simulink model "accBasedController_Simulation"  (R2020a)
settings: Solver=VariableStepAuto  StartTime=0  StopTime=20  FixedStep=0.001  RelTol=1e-3
values from neighbouring files (symbols this model uses):
  A = [0 0 5.53191489362 0 0 0 0 -107.82412766 0 221.276595745 0 1 ... (25 elements, 5x5)]    [CACu_ws.mat]    (also in SimulationParameters.m = [0 0 0 1 0 0;      0 0 0 0 1 0;      0 0 0 0 0 1;      -Ka/J; Simulation_ws.mat = [0 0 0 -118.993135011 5.87581816357 0 0 0 0 118.993135011 -1; abc_ws.mat = [0 0 0 1828.84460673 0 0 0 0 -1965.91569285 221.276595745 0 ; kalmanSS.m = [0 0 0 1 0 0;      0 0 0 0 1 0;      0 0 0 0 0 1;      -Ka/J)
  B = [1  0; 0  0; 0  0; 0  0; 0  19.2446808511]    [CACu_ws.mat]    (also in SimulationParameters.m = [zeros(3,control_dim); 1/Jh 0 0; 0 -1/Je 0; 0 0 N*KI/Ja]; Simulation_ws.mat = [0 0 0 22.8832951945 0 0 0 0 0 0 -1.12996503145 0 ... (18 el; abc_ws.mat = [1 0 0 0 0 0 0 0 -1.31799121269 0 0 0 ... (15 elements, 5x3); kalmanSS.m = [zeros(3,control_dim); 1/Jh 0 0; 0 -1/Je 0; 0 0 N*KI/Ja])
  C = [0 0 0 0 0 0 1 0 0 0 0 0 ... (25 elements, 5x5)]    [CACu_ws.mat]    (also in SimulationParameters.m = [zeros(sensor_dim,state_dim)]; Simulation_ws.mat = [-5.2 0 0 0 0 0 5.2 0 1 0 0 0 ... (36 elements, 6x6)]; abc_ws.mat; kalmanSS.m = [zeros(sensor_dim,state_dim)])
  CURRENT_MAX = 3.14    [CAC_ws.mat]    (also in CACu_ws.mat; SimulationParameters.m = 3.14159265359; Simulation_ws.mat = 3.14159265359; TransferFunctions.m = 3.14159265359)
  D = [1  0; 0  0; 0  0; 0  0; 0  0]    [CACu_ws.mat]    (also in SimulationParameters.m = zeros(sensor_dim, control_dim); Simulation_ws.mat = [0 0 0 0 0 0 0 0 0 0 0 0 ... (18 elements, 6x3)]; abc_ws.mat = [1 0 0 0 0 0 0 0 0 0 0 0 ... (15 elements, 5x3)]; kalmanSS.m = zeros(sensor_dim, control_dim))
  damping_d = 1.6    [CAC_ws.mat]    (also in CACu_ws.mat = 0.770835010154; abc_ws.mat = 0.770835010154; kalmanSSHumInput.m = 0.9; kalmanStateSpaceModellingHumInput.m = 0.9)
  dt = 0.001    [SimulationParameters.m]    (also in Simulation_ws.mat; TransferFunctions.m; kalmanSS.m; tests_analysis.m = 0.008)
  epos_Ki = 1.19    [CAC_ws.mat]    (also in CACu_ws.mat; TransferFunctions.m; abc_ws.mat; kalmanSSHumInput.m)
  epos_Kp = 11.9    [CAC_ws.mat]    (also in CACu_ws.mat; TransferFunctions.m; abc_ws.mat; kalmanSSHumInput.m)
  Fk = eye(state_dim) + A*dt + (A*dt)^2/prod(1:2) + (A*dt)^3/prod(1:3) + (A*dt)^4/prod(1:4)    [SimulationParameters.m]    (also in Simulation_ws.mat = [0.999940504052 2.93784973961e-06 5.41742100187e-11 -0.11899; kalmanSS.m)
  Gk = dt*(eye(state_dim) + A*dt/prod(1:2) + (A*dt)^2/prod(1:3) + (A*dt)^3/prod(1:4) +         (A*dt)^4/prod(1:5))*B    [SimulationParameters.m]    (also in Simulation_ws.mat = [1.14415341408e-05 5.60242006442e-12 0 0.0228828413715 2.240; kalmanSS.m = dt*(eye(state_dim) + A*dt/prod(1:2) + (A*dt)^2/prod(1:3) + ()
  I_zz = mass_scale*body_mass*(L_leg*r_zz)^2    (= 0.0437446334976)    [KneeJointParameters.m]    (also in SimulationParameters.m; Simulation_ws.mat; TransferFunctions.m; abc_ws.mat)
  Ja = 0.47    [CACu_ws.mat]    (also in SimulationParameters.m; Simulation_ws.mat; TransferFunctions.m; abc_ws.mat)
  Je = 0.94    [CACu_ws.mat]    (also in SimulationParameters.m = 0.88498313856; Simulation_ws.mat = 0.88498313856; TransferFunctions.m = 0.88498313856; abc_ws.mat = 0.7587304)
  Jh = 0.05    [CACu_ws.mat]    (also in SimulationParameters.m = 0.0437; Simulation_ws.mat = 0.0437; TransferFunctions.m = 0.0437; abc_ws.mat = 0.0437)
  Ka = 5.2    [CACu_ws.mat]    (also in SimulationParameters.m; Simulation_ws.mat; TransferFunctions.m = 6552; abc_ws.mat = 1387.6)
  KI = 0.0603    [CACu_ws.mat]    (also in SimulationParameters.m; Simulation_ws.mat; TransferFunctions.m; abc_ws.mat)
  Ks = 104    [CACu_ws.mat]    (also in SimulationParameters.m; Simulation_ws.mat; TransferFunctions.m; abc_ws.mat)
  Le = 0.4    [CACu_ws.mat]    (also in SimulationParameters.m = 0.432; Simulation_ws.mat = 0.432; TransferFunctions.m = 0.432; abc_ws.mat)
  N = 150    [CACu_ws.mat]    (also in SimulationParameters.m; Simulation_ws.mat; TransferFunctions.m; abc_ws.mat)
  Rk = eye(sensor_dim)    [kalmanStateSpaceModellingWithoutHum.m]
  sensor_dim = 5    [CACu_ws.mat]    (also in SimulationParameters.m = 6; Simulation_ws.mat = 6; abc_ws.mat; kalmanSS.m = 6)
  state_dim = 5    [CACu_ws.mat]    (also in SimulationParameters.m = 6; Simulation_ws.mat = 6; abc_ws.mat; kalmanSS.m = 6)
  stiffness_d = 1.04    [CAC_ws.mat]    (also in CACu_ws.mat = 14.0803237251; abc_ws.mat = 14.0803237251; kalmanSSHumInput.m = 3.874; kalmanStateSpaceModellingHumInput.m = 3.874)
  stiffness_lower = -20.9019922533    [CACu_ws.mat]    (also in abc_ws.mat; kalmanSSHumInput.m = -24.4873189611; kalmanStateSpaceModellingHumInput.m = -24.4873189611)
  Threaded_Ts = 0.001    [CAC_ws.mat]    (also in CACu_ws.mat; SimulationParameters.m; Simulation_ws.mat; abc_ws.mat)
  We = 19.6133    [CACu_ws.mat]    (also in SimulationParameters.m = 46.5037717323; Simulation_ws.mat = 46.5037717323; TransferFunctions.m = 46.5037717323; abc_ws.mat = 46.5037717323)
  zeta = 0.06    [SimulationParameters.m]    (also in Simulation_ws.mat; TransferFunctions.m; abc_ws.mat; kalmanSSHumInput.m = 0.01)
undefined symbols (not defined in the file or in its folder): A_kf, alpha, B_kf, C_kf, Continuous, D_kf, DiscIntNeverNeededParam, Discrete, gamma, k_bar, kf_ste_dim, nm_window, p_e_idx, p_m_idx, rho, sigma, Time, v_e_idx, v_h_idx, v_m_idx
libraries: simulink x23, dspstat3 x8, simulink_extras x5, ctrlSharedLib x2, dspsigops x2
(part 2 of 2)

== system accBasedController_Simulation/Secantes ==
  rms : Inport
  Trigger : TriggerPort  VariantControl=Variant
  Constant : Constant  Value=0.853
  Constant1 : Constant  Value=170
  Constant2 : Constant  Value=200
  Constant3 : Constant  Value=1.040
  Delay{,1..3} (4 alike) : Delay  DelayLength=1  InitialConditionSource=Input port
      settings: InputPortMap=u0,p4
  Divide : Product  Inputs=*/
  Product : Product
  Saturation : Saturate  UpperLimit=500  LowerLimit=0
  Sum : Sum  Inputs=+-
  Sum1 : Sum  Inputs=|-+
  Sum2 : Sum  Inputs=|+-
  Kp_new : Outport
  wires:
  rms/1 -> Delay3/1
  Constant/1 -> Delay/2
  Delay/1 -> Sum/2
  Product/1 -> Sum1/1
  Saturation/1 -> Delay1/1, Kp_new/1
  Constant1/1 -> Delay1/2
  Delay1/1 -> Delay2/1, Sum2/1, Sum1/2
  Divide/1 -> Product/2
  Sum/1 -> Divide/2
  Sum2/1 -> Divide/1
  Constant2/1 -> Delay2/2
  Constant3/1 -> Delay3/2
  Delay3/1 -> Delay/1, Sum/1, Product/1
  Delay2/1 -> Sum2/2
  Sum1/1 -> Saturation/1

== system accBasedController_Simulation/Subsystem ==
  x : Inport
  Constant12 : Constant  Value=1/dt
  Constant13 : Constant  Value=7
  Gain17 : Gain  Gain=1/(dt)
  LowPassFilter2p : Subsystem
  Sum : Sum  Inputs=|+-
  Unit Delay1 : UnitDelay  SampleTime=-1  HasFrameUpgradeWarning=on
  dot_x : Outport
  wires:
  Unit Delay1/1 -> Sum/2
  Sum/1 -> Gain17/1
  Gain17/1 -> LowPassFilter2p/1(sample)
  LowPassFilter2p/1(output) -> dot_x/1
  Constant12/1 -> LowPassFilter2p/3(sample_freq)
  x/1 -> Unit Delay1/1, Sum/1
  Constant13/1 -> LowPassFilter2p/2(cutoff_freq)

== system accBasedController_Simulation/Subsystem1 ==
  x : Inport
  Constant12 : Constant  Value=1/dt
  Constant13 : Constant  Value=7
  Gain17 : Gain  Gain=1/(dt)
  LowPassFilter2p : Subsystem
  Sum : Sum  Inputs=|+-
  Unit Delay1 : UnitDelay  SampleTime=-1  HasFrameUpgradeWarning=on
  dot_x : Outport
  wires:
  Constant13/1 -> LowPassFilter2p/2(cutoff_freq)
  x/1 -> Sum/1, Unit Delay1/1
  Constant12/1 -> LowPassFilter2p/3(sample_freq)
  LowPassFilter2p/1(output) -> dot_x/1
  Gain17/1 -> LowPassFilter2p/1(sample)
  Sum/1 -> Gain17/1
  Unit Delay1/1 -> Sum/2

== system accBasedController_Simulation/Subsystem2 ==
  x : Inport
  Constant12 : Constant  Value=1/dt
  Constant13 : Constant  Value=5
  Gain17 : Gain  Gain=1/(dt)
  LowPassFilter2p : Subsystem
  Sum : Sum  Inputs=|+-
  Unit Delay1 : UnitDelay  SampleTime=-1  HasFrameUpgradeWarning=on
  dot_x : Outport
  wires:
  Constant13/1 -> LowPassFilter2p/2(cutoff_freq)
  x/1 -> Sum/1, Unit Delay1/1
  Constant12/1 -> LowPassFilter2p/3(sample_freq)
  LowPassFilter2p/1(output) -> dot_x/1
  Gain17/1 -> LowPassFilter2p/1(sample)
  Sum/1 -> Gain17/1
  Unit Delay1/1 -> Sum/2

== system accBasedController_Simulation/UnitDelay ==
  In1 : Inport
  Unit Delay : UnitDelay  SampleTime=-1  HasFrameUpgradeWarning=on
  y : Outport  VectorParamsAs1DForOutWhenUnconnected=off
  wires:
  Unit Delay/1 -> y/1
  In1/1 -> Unit Delay/1

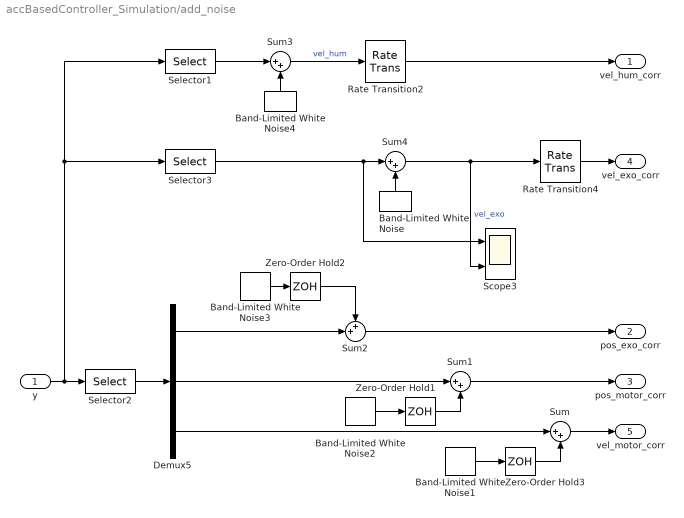
== system accBasedController_Simulation/add_noise ==
  y : Inport
  Band-Limited White Noise : simulink/Sources/Band-Limited White Noise  Cov=5.476e-6  Ts=dt  seed=[23341]  VectorParams1D=off
  Band-Limited White Noise1 : simulink/Sources/Band-Limited White Noise  Cov=1.096e-2  Ts=dt  seed=[23541]  VectorParams1D=off
  Band-Limited White Noise2 : simulink/Sources/Band-Limited White Noise  Cov=2.353e-6  Ts=dt  seed=[23543]  VectorParams1D=off
  Band-Limited White Noise3 : simulink/Sources/Band-Limited White Noise  Cov=9.412e-6  Ts=dt  seed=[87541]  VectorParams1D=off
  Band-Limited White Noise4 : simulink/Sources/Band-Limited White Noise  Cov=5.476e-6  Ts=dt  seed=[41236]  VectorParams1D=off
  Demux5 : Demux  Outputs=3
  Rate Transition2 : RateTransition  OutPortSampleTime=0.008
  Rate Transition4 : RateTransition  OutPortSampleTime=0.008
  Scope3 : Scope  NumInputPorts=2
  Selector1 : Selector  InputPortWidth=sensor_dim  IndexOptions=Index vector (dialog)  Indices=[v_h_idx]  OutputSizes=1
  Selector2 : Selector  InputPortWidth=sensor_dim  IndexOptions=Index vector (dialog)  Indices=[p_e_idx, p_m_idx, v_m_idx]  OutputSizes=1
  Selector3 : Selector  InputPortWidth=sensor_dim  IndexOptions=Index vector (dialog)  Indices=[v_e_idx]  OutputSizes=1
  Sum{,1,3..4} (4 alike) : Sum  Inputs=|++
  Sum2 : Sum  Inputs=++|
  Zero-Order Hold1 : ZeroOrderHold  SampleTime=dt
  Zero-Order Hold2 : ZeroOrderHold  SampleTime=dt
  Zero-Order Hold3 : ZeroOrderHold  SampleTime=dt
  vel_hum_corr : Outport
  pos_exo_corr : Outport  Port=2
  pos_motor_corr : Outport  Port=3
  vel_exo_corr : Outport  Port=4
  vel_motor_corr : Outport  Port=5
  wires:
  Selector2/1 -> Demux5/1
  Sum/1 -> vel_motor_corr/1
  Demux5/3 -> Sum/1
  Zero-Order Hold3/1 -> Sum/2
  y/1 -> Selector3/1, Selector1/1, Selector2/1
  Band-Limited White Noise1/1 -> Zero-Order Hold3/1
  Band-Limited White Noise2/1 -> Zero-Order Hold1/1
  Zero-Order Hold1/1 -> Sum1/2
  Sum1/1 -> pos_motor_corr/1
  Demux5/2 -> Sum1/1
  Band-Limited White Noise3/1 -> Zero-Order Hold2/1
  Sum2/1 -> pos_exo_corr/1
  Demux5/1 -> Sum2/2
  Zero-Order Hold2/1 -> Sum2/1
  Band-Limited White Noise4/1 -> Sum3/2
  Selector1/1 -> Sum3/1
  Sum3/1 -> Rate Transition2/1  "vel_hum"
  Rate Transition2/1 -> vel_hum_corr/1
  Selector3/1 -> Sum4/1, Scope3/1
  Sum4/1 -> Rate Transition4/1, Scope3/2  "vel_exo"
  Band-Limited White Noise/1 -> Sum4/2
  Rate Transition4/1 -> vel_exo_corr/1

== system accBasedController_Simulation/noise_resample_filtering ==
  vel_hum : Inport
  vel_exo : Inport  Port=2
  Band-Limited White Noise : simulink/Sources/Band-Limited White Noise  Cov=[dt*dt*0.3]  Ts=dt  seed=[23341]  VectorParams1D=off
  Band-Limited White Noise1 : simulink/Sources/Band-Limited White Noise  Cov=[dt*dt*0.3]  Ts=dt  seed=[41236]  VectorParams1D=off
  LowPassFilter2p : Subsystem
  LowPassFilter2p1 : Subsystem
  Rate Transition2 : RateTransition  OutPortSampleTime=0.008
  Rate Transition4 : RateTransition  OutPortSampleTime=0.008
  Scope3 : Scope  NumInputPorts=3
  Sum1 : Sum  Inputs=|++
  Sum2 : Sum  Inputs=|++
  XSENS_FC : Constant  Value=60
  XSENS_FC1 : Constant  Value=60
  XSENS_RATE : Constant  Value=120
  XSENS_RATE1 : Constant  Value=120
  ve_hum_filt : Outport
  vel_exo_filt : Outport  Port=2
  wires:
  vel_hum/1 -> Sum2/1
  XSENS_FC/1 -> LowPassFilter2p/2(cutoff_freq)
  LowPassFilter2p/1(output) -> ve_hum_filt/1  "vel_hum"
  XSENS_FC1/1 -> LowPassFilter2p1/2(cutoff_freq)
  Rate Transition4/1 -> LowPassFilter2p1/1(sample)
  vel_exo/1 -> Scope3/1, Sum1/1
  LowPassFilter2p1/1(output) -> vel_exo_filt/1, Scope3/3
  Sum2/1 -> Rate Transition2/1  "vel_hum"
  Sum1/1 -> Scope3/2, Rate Transition4/1  "vel_exo"
  Band-Limited White Noise1/1 -> Sum2/2
  Rate Transition2/1 -> LowPassFilter2p/1(sample)
  XSENS_RATE/1 -> LowPassFilter2p/3(sample_freq)
  Band-Limited White Noise/1 -> Sum1/2
  XSENS_RATE1/1 -> LowPassFilter2p1/3(sample_freq)

== system accBasedController_Simulation/update_Ki ==
  Kp_acc : Inport
  zeta : Inport  Port=2
  Bias : Bias  Bias=Je
  Gain2 : Gain  Gain=Ka
  Gain3 : Gain  Gain=2
  Product : Product
  Sqrt1 : Sqrt  SaturateOnIntegerOverflow=on
  Ki_acc : Outport
  wires:
  Bias/1 -> Gain2/1
  Gain2/1 -> Sqrt1/1
  Gain3/1 -> Ki_acc/1
  Kp_acc/1 -> Bias/1
  Sqrt1/1 -> Product/1
  Product/1 -> Gain3/1
  zeta/1 -> Product/2

== system accBasedController_Simulation/update_Kp ==
  w_n : Inport
  Constant : Constant  Value=Ka
  Divide : Product  Inputs=*/
  Gain1 : Gain  Gain=Je
  Square : Math  Operator=square  SaturateOnIntegerOverflow=on
  Sum : Sum  Inputs=|+-
  Kp_acc : Outport
  wires:
  Divide/1 -> Kp_acc/1
  Sum/1 -> Divide/1
  w_n/1 -> Square/1
  Constant/1 -> Sum/1
  Gain1/1 -> Sum/2
  Square/1 -> Divide/2, Gain1/1

== system accBasedController_Simulation/AccBasedController/A(z) ==
  In1 : Inport
  A(s) : TransferFcn  Numerator=[k_bar 0]  Denominator=[damping_d stiffness_d]
  Rate Transition1 : RateTransition  OutPortSampleTime=0.001
  Zero-Order Hold : ZeroOrderHold  SampleTime=-1
  Out1 : Outport
  wires:
  Zero-Order Hold/1 -> A(s)/1
  A(s)/1 -> Rate Transition1/1
  In1/1 -> Zero-Order Hold/1
  Rate Transition1/1 -> Out1/1

== system accBasedController_Simulation/AccBasedController/Filtering1 ==
  note: // get_filt_alpha - calculate a filter alpha
      | float AC_PID::get_filt_alpha(float filt_hz) const
      | {
      |     if (is_zero(filt_hz)) {
      |         return 1.0f;
      |     }
      |
      |     // calculate alpha
      |     float rc = 1 / (M_2PI * filt_hz);
      |     return _dt / (_dt + rc);
      | }
  note: e.g.:
      |
      | _target += get_filt_T_alpha() * (target - _target);
  new : Inport
  cutoff_freq [Hz] : Inport  Port=2
  reset_filter : Inport  Port=3
  dt : Inport  Port=4
  Constant6 : Constant
  Memory4 : Memory  InheritSampleTime=on
  Mux : Mux  Inputs=2
  Product5 : Product
  Subtract6 : Sum  Inputs=+-
  Subtract7 : Sum
  Switch : Switch  Criteria=u2 ~= 0
  Switch1 : Switch  Criteria=u2 ~= 0
  alpha : Fcn  Expr=u(1)/(u(1)+1/(2*pi*u(2)))
  filtered : Outport
  wires:
  Subtract7/1 -> Switch1/3
  Switch1/1 -> Memory4/1, filtered/1
  reset_filter/1 -> Switch1/2
  [alpha] -> Product5/1
  Switch/1 -> [alpha]
  Constant6/1 -> Switch/3
  new/1 -> Subtract6/1, Switch1/1
  Memory4/1 -> Subtract6/2, Subtract7/2
  Subtract6/1 -> Product5/2
  Product5/1 -> Subtract7/1
  Mux/1 -> alpha/1
  cutoff_freq [Hz]/1 -> Switch/2, Mux/2
  alpha/1 -> Switch/1
  dt/1 -> Mux/1

== system accBasedController_Simulation/AccBasedController/Filtering2 ==
  note: e.g.:
      |
      | _target += get_filt_T_alpha() * (target - _target);
  note: // get_filt_alpha - calculate a filter alpha
      | float AC_PID::get_filt_alpha(float filt_hz) const
      | {
      |     if (is_zero(filt_hz)) {
      |         return 1.0f;
      |     }
      |
      |     // calculate alpha
      |     float rc = 1 / (M_2PI * filt_hz);
      |     return _dt / (_dt + rc);
      | }
  new : Inport
  cutoff_freq [Hz] : Inport  Port=2
  reset_filter : Inport  Port=3
  dt : Inport  Port=4
  Constant6 : Constant
  Memory4 : Memory  InheritSampleTime=on
  Mux : Mux  Inputs=2
  Product5 : Product
  Subtract6 : Sum  Inputs=+-
  Subtract7 : Sum
  Switch : Switch  Criteria=u2 ~= 0
  Switch1 : Switch  Criteria=u2 ~= 0
  alpha : Fcn  Expr=u(1)/(u(1)+1/(2*pi*u(2)))
  filtered : Outport
  wires:
  dt/1 -> Mux/1
  alpha/1 -> Switch/1
  cutoff_freq [Hz]/1 -> Mux/2, Switch/2
  Mux/1 -> alpha/1
  Product5/1 -> Subtract7/1
  Subtract6/1 -> Product5/2
  Memory4/1 -> Subtract7/2, Subtract6/2
  new/1 -> Switch1/1, Subtract6/1
  Constant6/1 -> Switch/3
  Switch/1 -> [alpha]
  [alpha] -> Product5/1
  reset_filter/1 -> Switch1/2
  Switch1/1 -> filtered/1, Memory4/1
  Subtract7/1 -> Switch1/3

== system accBasedController_Simulation/AccBasedController/update_Ki ==
  Kp_acc : Inport
  Bias : Bias  Bias=Je
  Gain2 : Gain  Gain=Ka
  Gain3 : Gain  Gain=2*zeta
  Sqrt1 : Sqrt  SaturateOnIntegerOverflow=on
  Ki_acc : Outport
  wires:
  Sqrt1/1 -> Gain3/1
  Bias/1 -> Gain2/1
  Gain2/1 -> Sqrt1/1
  Gain3/1 -> Ki_acc/1
  Kp_acc/1 -> Bias/1

== system accBasedController_Simulation/AccBasedController/update_Kp ==
  w_n_sq : Inport
  Constant : Constant  Value=Ka
  Divide : Product  Inputs=*/
  Gain1 : Gain  Gain=Je
  Sum : Sum  Inputs=|+-
  Kp_acc : Outport
  wires:
  Divide/1 -> Kp_acc/1
  Sum/1 -> Divide/1
  w_n_sq/1 -> Divide/2, Gain1/1
  Constant/1 -> Sum/1
  Gain1/1 -> Sum/2

== system accBasedController_Simulation/AccBasedController/w_n_desired ==
  KneePosition : Inport
  Gain2 : Gain  Gain=1/I_zz
  k0 : Bias  Bias=110.0
  k1 : Gain  Gain=169.3
  w_n_sq : Outport
  wires:
  KneePosition/1 -> k1/1
  k1/1 -> k0/1
  Gain2/1 -> w_n_sq/1
  k0/1 -> Gain2/1  "K_j"

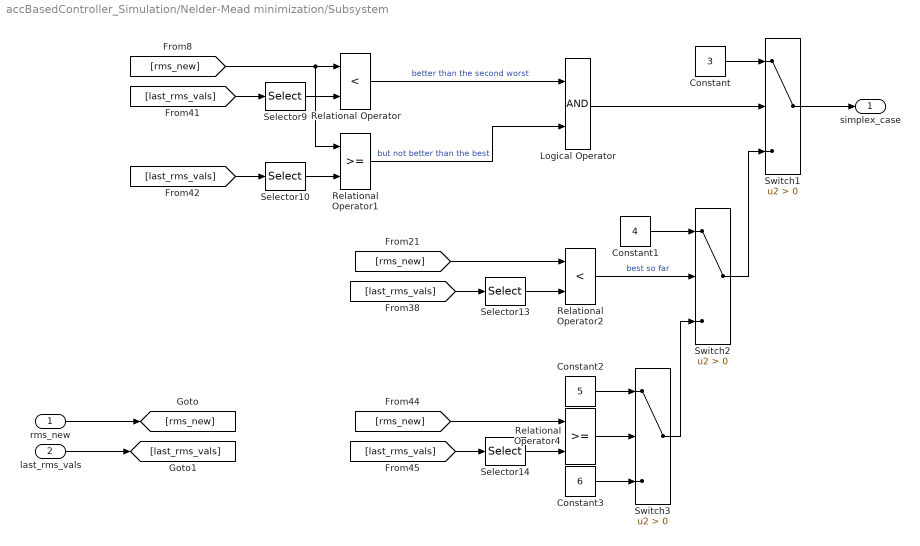
== system accBasedController_Simulation/Nelder-Mead minimization/Subsystem ==
  rms_new : Inport
  last_rms_vals : Inport  Port=2
  Constant : Constant  Value=3
  Constant1 : Constant  Value=4
  Constant2 : Constant  Value=5
  Constant3 : Constant  Value=6
  Logical Operator : Logic  AllPortsSameDT=off  OutDataTypeStr=boolean
  Relational Operator : RelationalOperator  Operator=<  OutDataTypeStr=boolean  RndMeth=Simplest
  Relational Operator1 : RelationalOperator  OutDataTypeStr=boolean  RndMeth=Simplest
  Relational Operator2 : RelationalOperator  Operator=<  OutDataTypeStr=boolean  RndMeth=Simplest
  Relational Operator4 : RelationalOperator  OutDataTypeStr=boolean  RndMeth=Simplest
  Selector10 : Selector  InputPortWidth=3  IndexOptions=Index vector (dialog)  Indices=[1]  OutputSizes=1
  Selector13 : Selector  InputPortWidth=3  IndexOptions=Index vector (dialog)  Indices=[1]  OutputSizes=1
  Selector14 : Selector  InputPortWidth=3  IndexOptions=Index vector (dialog)  Indices=[2]  OutputSizes=1
  Selector9 : Selector  InputPortWidth=3  IndexOptions=Index vector (dialog)  Indices=[2]  OutputSizes=1
  Switch1 : Switch  Criteria=u2 > Threshold
  Switch2 : Switch  Criteria=u2 > Threshold
  Switch3 : Switch  Criteria=u2 > Threshold
  simplex_case : Outport
  wires:
  Switch2/1 -> Switch1/3
  Selector10/1 -> Relational Operator1/2
  [last_rms_vals] -> Selector14/1
  Constant1/1 -> Switch2/1
  Constant3/1 -> Switch3/3
  Logical Operator/1 -> Switch1/2
  Relational Operator4/1 -> Switch3/2
  [last_rms_vals] -> Selector9/1
  Constant2/1 -> Switch3/1
  [last_rms_vals] -> Selector10/1
  [rms_new] -> Relational Operator4/1
  Switch1/1 -> simplex_case/1
  Switch3/1 -> Switch2/3
  Relational Operator2/1 -> Switch2/2  "best so far"
  [rms_new] -> Relational Operator1/1, Relational Operator/1
  Selector14/1 -> Relational Operator4/2
  Relational Operator1/1 -> Logical Operator/2  "but not better than the best"
  Constant/1 -> Switch1/1
  Relational Operator/1 -> Logical Operator/1  "better than the second worst"
  [last_rms_vals] -> Selector13/1
  [rms_new] -> Relational Operator2/1
  Selector9/1 -> Relational Operator/2
  Selector13/1 -> Relational Operator2/2
  rms_new/1 -> [rms_new]
  last_rms_vals/1 -> [last_rms_vals]

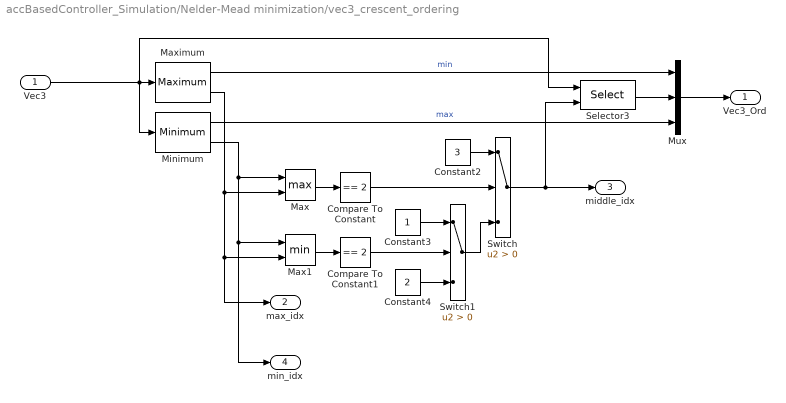
== system accBasedController_Simulation/Nelder-Mead minimization/vec3_crescent_ordering ==
  Vec3 : Inport
  Compare To Constant : simulink/Logic and Bit Operations/Compare To Constant  relop===  const=2  OutDataTypeStr=boolean
  Compare To Constant1 : simulink/Logic and Bit Operations/Compare To Constant  relop===  const=2  OutDataTypeStr=boolean
  Constant2 : Constant  Value=3
  Constant3 : Constant
  Constant4 : Constant  Value=2
  Max : MinMax  Function=max  Inputs=2
  Max1 : MinMax  Inputs=2
  Maximum : dspstat3/Maximum  operation=maximum  fcn=Value and Index  indexBase=One  operateOver=Each column  Dimension=1  InputProcessing=Columns as channels (frame based)  reset=None  roiEnable=off  roiType=Rectangles  roiPortion=Entire ROI  roiOutput=Individual statistics for each ROI  roiFlag=off  roundingMode=Floor  overflowMode=off  accumDataTypeStr=Inherit: Same as product output  accumLastDataTypeStr=Inherit: Same as product output
  Minimum : dspstat3/Minimum  operation=minimum  fcn=Value and Index  indexBase=One  operateOver=Each column  Dimension=1  InputProcessing=Columns as channels (frame based)  reset=None  roiEnable=off  roiType=Rectangles  roiPortion=Entire ROI  roiOutput=Individual statistics for each ROI  roiFlag=off  roundingMode=Floor  overflowMode=off
      settings: SourceProductBaseCode=DS
  Mux : Mux  Inputs=3
  Selector3 : Selector  InputPortWidth=3  IndexOptions=Index vector (port)  Indices=[1 3]  OutputSizes=1
  Switch : Switch  Criteria=u2 > Threshold
  Switch1 : Switch  Criteria=u2 > Threshold
  Vec3_Ord : Outport
  max_idx : Outport  Port=2
  middle_idx : Outport  Port=3
  min_idx : Outport  Port=4
  wires:
  Constant3/1 -> Switch1/1
  Minimum/2 -> Max/1, min_idx/1, Max1/1
  Vec3/1 -> Minimum/1, Maximum/1, Selector3/1
  Constant2/1 -> Switch/1
  Switch/1 -> middle_idx/1, Selector3/2
  Max1/1 -> Compare To Constant1/1
  Maximum/2 -> Max1/2, max_idx/1, Max/2
  Constant4/1 -> Switch1/3
  Max/1 -> Compare To Constant/1
  Compare To Constant1/1 -> Switch1/2
  Switch1/1 -> Switch/3
  Compare To Constant/1 -> Switch/2
  Mux/1 -> Vec3_Ord/1
  Minimum/1 -> Mux/3  "max"
  Selector3/1 -> Mux/2
  Maximum/1 -> Mux/1  "min"

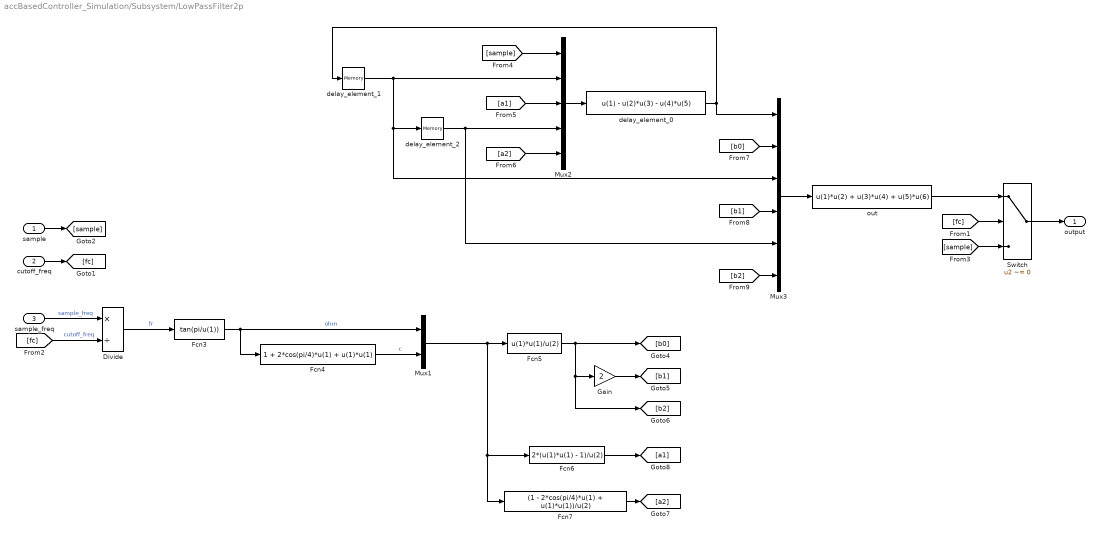
== system accBasedController_Simulation/Subsystem/LowPassFilter2p ==
  sample : Inport
  cutoff_freq : Inport  Port=2
  sample_freq : Inport  Port=3
  Divide : Product  Inputs=*/
  Fcn3 : Fcn  Expr=tan(pi/u(1))
  Fcn4 : Fcn  Expr=1 + 2*cos(pi/4)*u(1) + u(1)*u(1)
  Fcn5 : Fcn  Expr=u(1)*u(1)/u(2)
  Fcn6 : Fcn  Expr=2*(u(1)*u(1) - 1)/u(2)
  Fcn7 : Fcn  Expr=(1 - 2*cos(pi/4)*u(1) + u(1)*u(1))/u(2)
  Gain : Gain  Gain=2
  Mux1 : Mux  Inputs=2
  Mux2 : Mux  Inputs=5
  Mux3 : Mux  Inputs=6
  Switch : Switch  Criteria=u2 ~= 0
  delay_element_0 : Fcn  Expr=u(1) - u(2)*u(3) - u(4)*u(5)
  delay_element_1 : Memory  InheritSampleTime=on
  delay_element_2 : Memory  InheritSampleTime=on
  out : Fcn  Expr=u(1)*u(2) + u(3)*u(4) + u(5)*u(6)
  output : Outport
  wires:
  Switch/1 -> output/1
  cutoff_freq/1 -> [fc]
  [fc] -> Switch/2
  sample_freq/1 -> Divide/1  "sample_freq"
  [fc] -> Divide/2  "cutoff_freq"
  Divide/1 -> Fcn3/1  "fr"
  Mux1/1 -> Fcn7/1, Fcn6/1, Fcn5/1
  Fcn3/1 -> Mux1/1, Fcn4/1  "ohm"
  Fcn4/1 -> Mux1/2  "c"
  Fcn5/1 -> [b0], [b2], Gain/1
  Gain/1 -> [b1]
  Fcn6/1 -> [a1]
  Fcn7/1 -> [a2]
  sample/1 -> [sample]
  [sample] -> Switch/3
  delay_element_1/1 -> delay_element_2/1, Mux3/3, Mux2/2
  [sample] -> Mux2/1
  Mux2/1 -> delay_element_0/1
  [a1] -> Mux2/3
  delay_element_2/1 -> Mux2/4, Mux3/5
  [a2] -> Mux2/5
  out/1 -> Switch/1
  delay_element_0/1 -> delay_element_1/1, Mux3/1
  [b0] -> Mux3/2
  [b1] -> Mux3/4
  [b2] -> Mux3/6
  Mux3/1 -> out/1

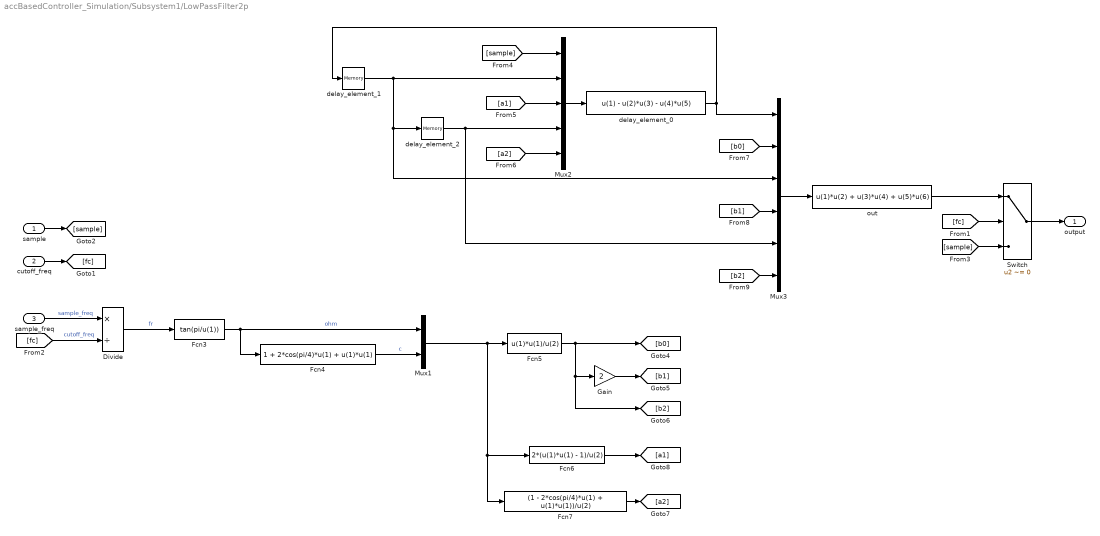
== system accBasedController_Simulation/Subsystem1/LowPassFilter2p ==
  sample : Inport
  cutoff_freq : Inport  Port=2
  sample_freq : Inport  Port=3
  Divide : Product  Inputs=*/
  Fcn3 : Fcn  Expr=tan(pi/u(1))
  Fcn4 : Fcn  Expr=1 + 2*cos(pi/4)*u(1) + u(1)*u(1)
  Fcn5 : Fcn  Expr=u(1)*u(1)/u(2)
  Fcn6 : Fcn  Expr=2*(u(1)*u(1) - 1)/u(2)
  Fcn7 : Fcn  Expr=(1 - 2*cos(pi/4)*u(1) + u(1)*u(1))/u(2)
  Gain : Gain  Gain=2
  Mux1 : Mux  Inputs=2
  Mux2 : Mux  Inputs=5
  Mux3 : Mux  Inputs=6
  Switch : Switch  Criteria=u2 ~= 0
  delay_element_0 : Fcn  Expr=u(1) - u(2)*u(3) - u(4)*u(5)
  delay_element_1 : Memory  InheritSampleTime=on
  delay_element_2 : Memory  InheritSampleTime=on
  out : Fcn  Expr=u(1)*u(2) + u(3)*u(4) + u(5)*u(6)
  output : Outport
  wires:
  Mux3/1 -> out/1
  [b2] -> Mux3/6
  [b1] -> Mux3/4
  [b0] -> Mux3/2
  delay_element_0/1 -> Mux3/1, delay_element_1/1
  out/1 -> Switch/1
  [a2] -> Mux2/5
  delay_element_2/1 -> Mux3/5, Mux2/4
  [a1] -> Mux2/3
  Mux2/1 -> delay_element_0/1
  [sample] -> Mux2/1
  delay_element_1/1 -> Mux2/2, Mux3/3, delay_element_2/1
  [sample] -> Switch/3
  sample/1 -> [sample]
  Fcn7/1 -> [a2]
  Fcn6/1 -> [a1]
  Gain/1 -> [b1]
  Fcn5/1 -> Gain/1, [b2], [b0]
  Fcn4/1 -> Mux1/2  "c"
  Fcn3/1 -> Fcn4/1, Mux1/1  "ohm"
  Mux1/1 -> Fcn5/1, Fcn6/1, Fcn7/1
  Divide/1 -> Fcn3/1  "fr"
  [fc] -> Divide/2  "cutoff_freq"
  sample_freq/1 -> Divide/1  "sample_freq"
  [fc] -> Switch/2
  cutoff_freq/1 -> [fc]
  Switch/1 -> output/1

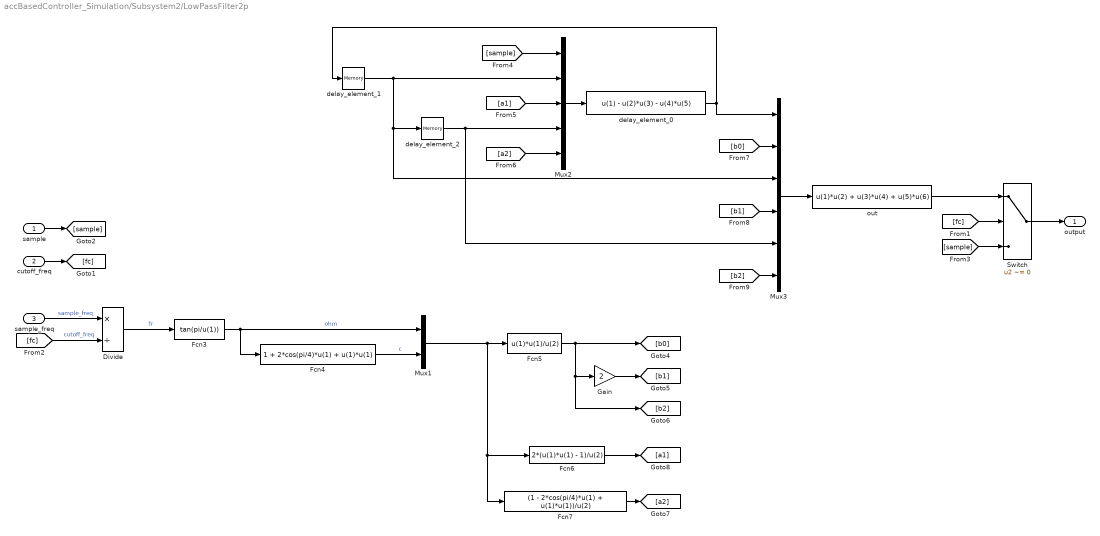
== system accBasedController_Simulation/Subsystem2/LowPassFilter2p ==
  sample : Inport
  cutoff_freq : Inport  Port=2
  sample_freq : Inport  Port=3
  Divide : Product  Inputs=*/
  Fcn3 : Fcn  Expr=tan(pi/u(1))
  Fcn4 : Fcn  Expr=1 + 2*cos(pi/4)*u(1) + u(1)*u(1)
  Fcn5 : Fcn  Expr=u(1)*u(1)/u(2)
  Fcn6 : Fcn  Expr=2*(u(1)*u(1) - 1)/u(2)
  Fcn7 : Fcn  Expr=(1 - 2*cos(pi/4)*u(1) + u(1)*u(1))/u(2)
  Gain : Gain  Gain=2
  Mux1 : Mux  Inputs=2
  Mux2 : Mux  Inputs=5
  Mux3 : Mux  Inputs=6
  Switch : Switch  Criteria=u2 ~= 0
  delay_element_0 : Fcn  Expr=u(1) - u(2)*u(3) - u(4)*u(5)
  delay_element_1 : Memory  InheritSampleTime=on
  delay_element_2 : Memory  InheritSampleTime=on
  out : Fcn  Expr=u(1)*u(2) + u(3)*u(4) + u(5)*u(6)
  output : Outport
  wires:
  Mux3/1 -> out/1
  [b2] -> Mux3/6
  [b1] -> Mux3/4
  [b0] -> Mux3/2
  delay_element_0/1 -> Mux3/1, delay_element_1/1
  out/1 -> Switch/1
  [a2] -> Mux2/5
  delay_element_2/1 -> Mux3/5, Mux2/4
  [a1] -> Mux2/3
  Mux2/1 -> delay_element_0/1
  [sample] -> Mux2/1
  delay_element_1/1 -> Mux2/2, Mux3/3, delay_element_2/1
  [sample] -> Switch/3
  sample/1 -> [sample]
  Fcn7/1 -> [a2]
  Fcn6/1 -> [a1]
  Gain/1 -> [b1]
  Fcn5/1 -> Gain/1, [b2], [b0]
  Fcn4/1 -> Mux1/2  "c"
  Fcn3/1 -> Fcn4/1, Mux1/1  "ohm"
  Mux1/1 -> Fcn5/1, Fcn6/1, Fcn7/1
  Divide/1 -> Fcn3/1  "fr"
  [fc] -> Divide/2  "cutoff_freq"
  sample_freq/1 -> Divide/1  "sample_freq"
  [fc] -> Switch/2
  cutoff_freq/1 -> [fc]
  Switch/1 -> output/1

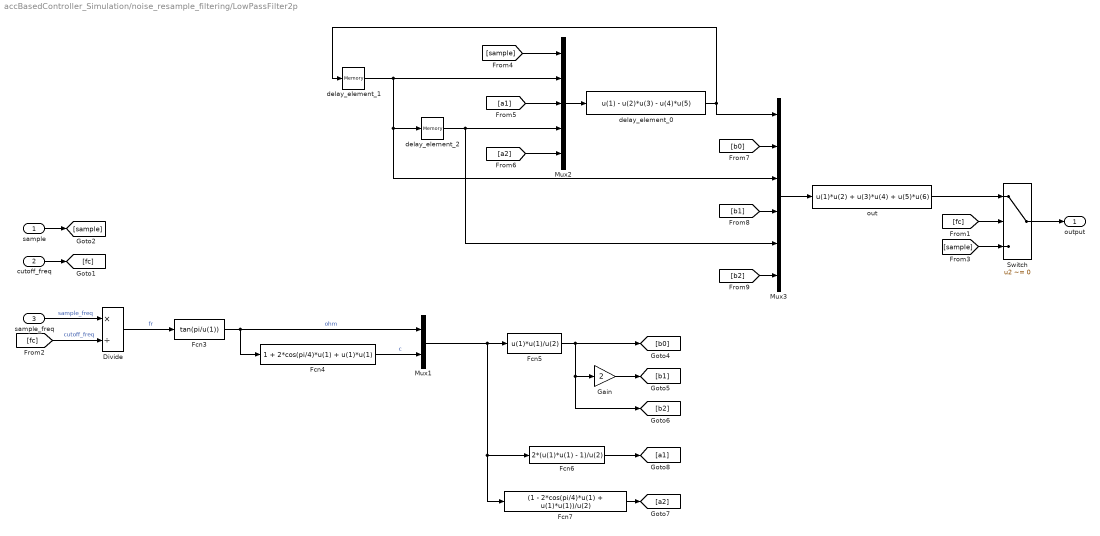
== system accBasedController_Simulation/noise_resample_filtering/LowPassFilter2p ==
  sample : Inport
  cutoff_freq : Inport  Port=2
  sample_freq : Inport  Port=3
  Divide : Product  Inputs=*/
  Fcn3 : Fcn  Expr=tan(pi/u(1))
  Fcn4 : Fcn  Expr=1 + 2*cos(pi/4)*u(1) + u(1)*u(1)
  Fcn5 : Fcn  Expr=u(1)*u(1)/u(2)
  Fcn6 : Fcn  Expr=2*(u(1)*u(1) - 1)/u(2)
  Fcn7 : Fcn  Expr=(1 - 2*cos(pi/4)*u(1) + u(1)*u(1))/u(2)
  Gain : Gain  Gain=2
  Mux1 : Mux  Inputs=2
  Mux2 : Mux  Inputs=5
  Mux3 : Mux  Inputs=6
  Switch : Switch  Criteria=u2 ~= 0
  delay_element_0 : Fcn  Expr=u(1) - u(2)*u(3) - u(4)*u(5)
  delay_element_1 : Memory  InheritSampleTime=on
  delay_element_2 : Memory  InheritSampleTime=on
  out : Fcn  Expr=u(1)*u(2) + u(3)*u(4) + u(5)*u(6)
  output : Outport
  wires:
  Switch/1 -> output/1
  cutoff_freq/1 -> [fc]
  [fc] -> Switch/2
  sample_freq/1 -> Divide/1  "sample_freq"
  [fc] -> Divide/2  "cutoff_freq"
  Divide/1 -> Fcn3/1  "fr"
  Mux1/1 -> Fcn7/1, Fcn6/1, Fcn5/1
  Fcn3/1 -> Mux1/1, Fcn4/1  "ohm"
  Fcn4/1 -> Mux1/2  "c"
  Fcn5/1 -> [b0], [b2], Gain/1
  Gain/1 -> [b1]
  Fcn6/1 -> [a1]
  Fcn7/1 -> [a2]
  sample/1 -> [sample]
  [sample] -> Switch/3
  delay_element_1/1 -> delay_element_2/1, Mux3/3, Mux2/2
  [sample] -> Mux2/1
  Mux2/1 -> delay_element_0/1
  [a1] -> Mux2/3
  delay_element_2/1 -> Mux2/4, Mux3/5
  [a2] -> Mux2/5
  out/1 -> Switch/1
  delay_element_0/1 -> delay_element_1/1, Mux3/1
  [b0] -> Mux3/2
  [b1] -> Mux3/4
  [b2] -> Mux3/6
  Mux3/1 -> out/1

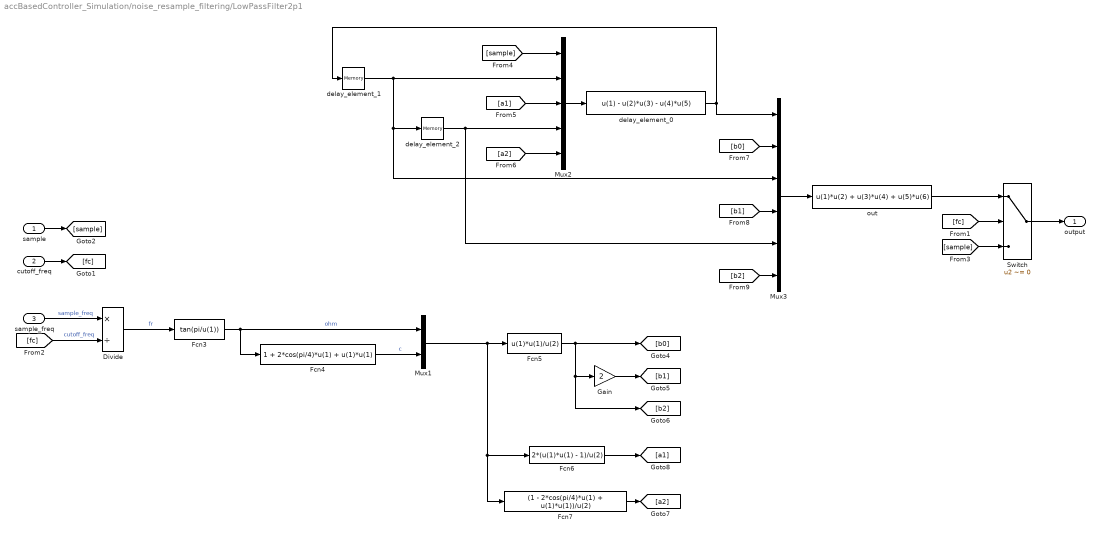
== system accBasedController_Simulation/noise_resample_filtering/LowPassFilter2p1 ==
  sample : Inport
  cutoff_freq : Inport  Port=2
  sample_freq : Inport  Port=3
  Divide : Product  Inputs=*/
  Fcn3 : Fcn  Expr=tan(pi/u(1))
  Fcn4 : Fcn  Expr=1 + 2*cos(pi/4)*u(1) + u(1)*u(1)
  Fcn5 : Fcn  Expr=u(1)*u(1)/u(2)
  Fcn6 : Fcn  Expr=2*(u(1)*u(1) - 1)/u(2)
  Fcn7 : Fcn  Expr=(1 - 2*cos(pi/4)*u(1) + u(1)*u(1))/u(2)
  Gain : Gain  Gain=2
  Mux1 : Mux  Inputs=2
  Mux2 : Mux  Inputs=5
  Mux3 : Mux  Inputs=6
  Switch : Switch  Criteria=u2 ~= 0
  delay_element_0 : Fcn  Expr=u(1) - u(2)*u(3) - u(4)*u(5)
  delay_element_1 : Memory  InheritSampleTime=on
  delay_element_2 : Memory  InheritSampleTime=on
  out : Fcn  Expr=u(1)*u(2) + u(3)*u(4) + u(5)*u(6)
  output : Outport
  wires:
  Mux3/1 -> out/1
  [b2] -> Mux3/6
  [b1] -> Mux3/4
  [b0] -> Mux3/2
  delay_element_0/1 -> Mux3/1, delay_element_1/1
  out/1 -> Switch/1
  [a2] -> Mux2/5
  delay_element_2/1 -> Mux3/5, Mux2/4
  [a1] -> Mux2/3
  Mux2/1 -> delay_element_0/1
  [sample] -> Mux2/1
  delay_element_1/1 -> Mux2/2, Mux3/3, delay_element_2/1
  [sample] -> Switch/3
  sample/1 -> [sample]
  Fcn7/1 -> [a2]
  Fcn6/1 -> [a1]
  Gain/1 -> [b1]
  Fcn5/1 -> Gain/1, [b2], [b0]
  Fcn4/1 -> Mux1/2  "c"
  Fcn3/1 -> Fcn4/1, Mux1/1  "ohm"
  Mux1/1 -> Fcn5/1, Fcn6/1, Fcn7/1
  Divide/1 -> Fcn3/1  "fr"
  [fc] -> Divide/2  "cutoff_freq"
  sample_freq/1 -> Divide/1  "sample_freq"
  [fc] -> Switch/2
  cutoff_freq/1 -> [fc]
  Switch/1 -> output/1
